simulink model "InvertedPendulumPolePlacement_REV0"  (R2018a)
settings: Solver=VariableStepAuto  StartTime=0.0  StopTime=10.0  RelTol=1e-3
values from neighbouring files (symbols this model uses):
  Ac = [0 1 0 0 ... (first row only)    [BasicModelParameters.m]    (also in ControllerDesign_REV0.m; FurutaPendulum.m = [0 1 0 0; 0 0 -a23 0; 0 0 0 1; 0 0 a43 0]; InvertedPendulumStepResponse.m)
  Bc = transpose([0 b21 0 -b41])    [BasicModelParameters.m]    (also in ControllerDesign_REV0.m; FurutaPendulum.m = [0; b21; 0; -b41]; InvertedPendulumStepResponse.m)
  Cc = [1 0 0 0 ... (first row only)    [BasicModelParameters.m]    (also in ControllerDesign_REV0.m; FurutaPendulum.m = [1 0 0 0; 0 0 1 0]; InvertedPendulumStepResponse.m)
  Dc = [0 ... (first row only)    [BasicModelParameters.m]    (also in ControllerDesign_REV0.m; FurutaPendulum.m = [0; 0]; InvertedPendulumStepResponse.m)
  k_DC = evalfr(Hcl_s(1), 0)    [PolePlacementDesign_REV0.m]
  K_s = place(Ac,Bc,Pcld_s)    [FurutaPendulum.m]    (also in PolePlacementDesign_REV0.m = place(Ac, Bc, Pcld_s))
  Ts = 0.0017    [ControllerDesign_REV0.m]    (also in InvertedPendulum.m; InvertedPendulumStepResponse.m; PolePlacementDesign_REV0.m = 0.01)
settings Model: Creator=Jack  LastModifiedBy=Jack

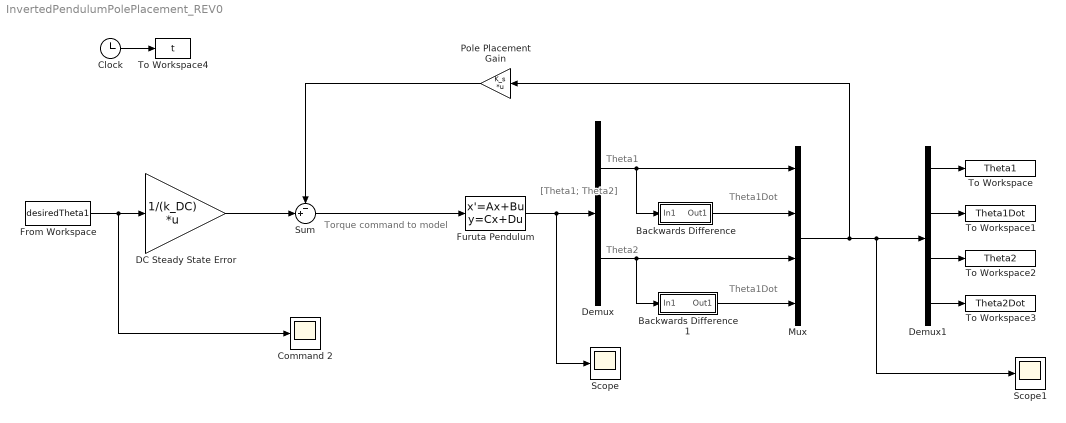
== system InvertedPendulumPolePlacement_REV0 ==
  note: Theta1Dot
  note: Theta1
  note: [Theta1;
      | Theta2]
  note: Torque command to model
  note: Theta2
  note: Theta1Dot
  "Backwards Difference " : Subsystem
  Backwards Difference 1 : Subsystem
  Clock : Clock
  Command 2 : Scope
  DC Steady State Error : Gain  Gain=1/(k_DC)  Multiplication=Matrix(K*u)
  Demux : Demux  Outputs=2
  Demux1 : Demux
  From Workspace : FromWorkspace  VariableName=desiredTheta1  SampleTime=0
  Furuta Pendulum : StateSpace  A=Ac  B=Bc  C=Cc  D=Dc  InitialCondition=[0; 0; 0.05; 0]  ContinuousStateAttributes='Theta'
  Mux : Mux
  Pole Placement Gain : Gain  Gain=K_s  Multiplication=Matrix(K*u)
  Scope : Scope
  Scope1 : Scope
  Sum : Sum  Inputs=-+|
  To Workspace : ToWorkspace  VariableName=Theta1  SampleTime=-1
  To Workspace1 : ToWorkspace  VariableName=Theta1Dot  SampleTime=-1
  To Workspace2 : ToWorkspace  VariableName=Theta2  SampleTime=-1
  To Workspace3 : ToWorkspace  VariableName=Theta2Dot  SampleTime=-1
  To Workspace4 : ToWorkspace  VariableName=t  SampleTime=-1
      settings: Save2DSignal=2-D array (concatenate along first dimension)
  wires:
  From Workspace/1 -> Command 2/1, DC Steady State Error/1
  DC Steady State Error/1 -> Sum/2
  Sum/1 -> Furuta Pendulum/1
  Pole Placement Gain/1 -> Sum/1
  Furuta Pendulum/1 -> Scope/1, Demux/1
  Demux/1 -> "Backwards Difference "/1(In1), Mux/1
  "Backwards Difference "/1(Out1) -> Mux/2
  Backwards Difference 1/1(Out1) -> Mux/4
  Demux/2 -> Backwards Difference 1/1(In1), Mux/3
  Mux/1 -> Scope1/1, Demux1/1, Pole Placement Gain/1
  Demux1/1 -> To Workspace/1
  Demux1/4 -> To Workspace3/1
  Demux1/3 -> To Workspace2/1
  Demux1/2 -> To Workspace1/1
  Clock/1 -> To Workspace4/1

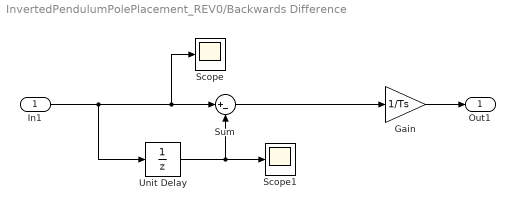
== system InvertedPendulumPolePlacement_REV0/Backwards Difference  ==
  In1 : Inport
  Gain : Gain  Gain=1/Ts
  Scope : Scope
  Scope1 : Scope
  Sum : Sum  Inputs=|+-
  Unit Delay : UnitDelay  SampleTime=Ts
  Out1 : Outport
  wires:
  In1/1 -> Unit Delay/1, Scope/1, Sum/1
  Unit Delay/1 -> Scope1/1, Sum/2
  Sum/1 -> Gain/1
  Gain/1 -> Out1/1

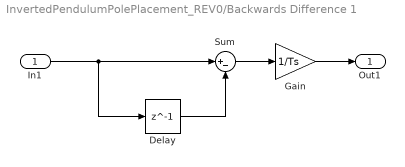
== system InvertedPendulumPolePlacement_REV0/Backwards Difference 1 ==
  In1 : Inport
  Delay : Delay  DelayLength=1
  Gain : Gain  Gain=1/Ts
  Sum : Sum  Inputs=|+-
  Out1 : Outport
  wires:
  In1/1 -> Sum/1, Delay/1
  Delay/1 -> Sum/2
  Sum/1 -> Gain/1
  Gain/1 -> Out1/1
